simulink model "difdriveintegration"  (R2022b)
settings: Solver=VariableStepAuto  StartTime=0.0  StopTime=10  RelTol=1e-3
InitFcn:
  | r = 0.1
  | L = 0.5
settings Model: Creator=Jordan  LastModifiedBy=Jordan

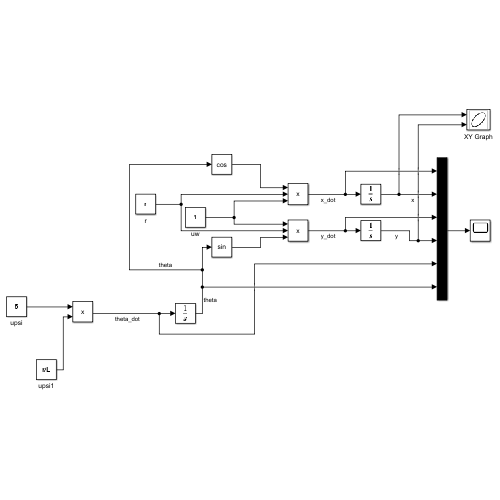
[thumbnail: Simulink's stored preview of the top-level diagram]
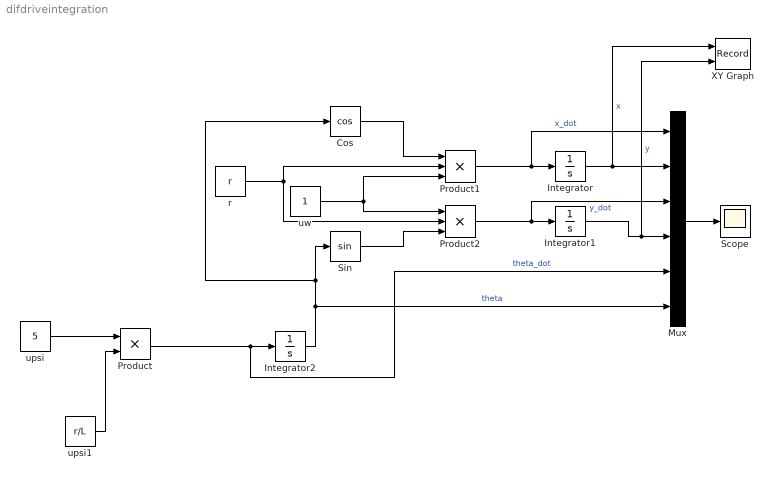
== system difdriveintegration ==
  Cos : Trigonometry  Operator=cos
  Integrator : Integrator
  Integrator1 : Integrator
  Integrator2 : Integrator
  Mux : Mux  Inputs=6
  Product : Product
  Product1 : Product  Inputs=3
  Product2 : Product  Inputs=3
  Scope : Scope
  Sin : Trigonometry
  XY Graph : Record  FileSettingsInternal="{\"entries\":[{\"content\":{\"excelSettings\":{\"content\":{},\"type\":\"Streamout.ExcelSettings\"}},\"type\":\"Streamout.FileSettingStorage\",\"uuid\":\"2d7a5891-e8f7-4a24-a04d-ef72669cf435\"}],\"packageUris\":[\"http://schema.mathworks.com/mf0/streamout_blocks/R2020a\"],\"version\":\"1.0\"}"  Layout=[1 1]  SignalsInternal="{\"entries\":[{\"content\":{\"signals\":[{\"content\":{\"blockPath\":[\"untitled/XY Graph\"],\"channel\":[],\"dimensions\":[1],\"domain\":\"untitled/XY Graph\",\"lineColor\":\"#a2142f\",\"plots\":[1],\"port\":1,\"sid\":[\"\"],\"signalID\":170,\"signalName\":\"x\"},\"type\":\"RecordBlkView.Signal\",\"uuid\":\"1ee0a7eb-6eb6-43d4-87cb-68a379b61913\"},{\"content\":{\"blockPath\":[\"untitled/XY Graph\"],\"channel\":[],\"dimensions\":[1],\"domain\":\"untitled/XY Graph\",\"lineColor\":\"#139fff\",\"plots\":[1],\"port\":2,\"sid\":[\"\"],\"signalID\":174,\"signalName\":\"y\"},\"type\":\"RecordBlkView.Signal\",\"uuid\":\"58b255e7-f1e4-4212-8ee9-47a1400495a9\"}]},\"type\":\"RecordBlkView.InputSignals\",\"uuid\":\"1fc7c7c5-e227-4a1c-a976-7326235ed89c\"}],\"packageUris\":[\"http://schema.mathworks.com/mf0/streamout_blocks/R2020a\"],\"version\":\"1.0\"}"  VisualizationBindings="{\"xyplotplugin\":{\"info\":[{\"series\":[{\"bindingParametersList\":[{\"parameter\":\"X-Axis\",\"signalID\":170,\"signalName\":\"x\"},{\"parameter\":\"Y-Axis\",\"signalID\":174,\"signalName\":\"y\"}],\"seriesID\":41152}],\"subplotID\":1}]}}"  CompatibilityTag=XY
  r : Constant  Value=r
  upsi : Constant  Value=5
  upsi1 : Constant  Value=r/L
  uw : Constant
  wires:
  upsi/1 -> Product/1
  upsi1/1 -> Product/2
  Product/1 -> Mux/5, Integrator2/1  "theta_dot"
  uw/1 -> Product2/1, Product1/3
  r/1 -> Product1/2, Product2/2
  Cos/1 -> Product1/1
  Sin/1 -> Product2/3
  Integrator2/1 -> Mux/6, Cos/1, Sin/1  "theta"
  Product2/1 -> Mux/3, Integrator1/1  "y_dot"
  Product1/1 -> Mux/1, Integrator/1  "x_dot"
  Integrator/1 -> XY Graph/1, Mux/2  "x"
  Integrator1/1 -> XY Graph/2, Mux/4  "y"
  Mux/1 -> Scope/1
